simulink model "VirtualMotoTemplate"  (R2025b)
settings: Solver=daessc  StartTime=0  StopTime=2474  FixedStep=.001  RelTol=1e-2  EnableMultiTasking=on
StopFcn:
  | %toc
undefined symbols (not defined in the file): AccelOvrCmd, CtrlTcuInitGear, DecelOvrCmd, Disabled, DriverPreviewDist, EnblAccelOvr, EnblDecelCmd, EnblSteerCmd, EnvAbsPrs, EnvAirTemp, EnvGrvty, EnvNomFrictionScaling, EnvNominalGrade, EnvWindVelX, EnvWindVelY, EnvWindVelZ, FTP75, MotoFrmInert, MotoFrmLngth, MotoFrmMass, MotoLowrFrntFrkMass, MotoRearArmLngth, MotoRearArmMass, MotoUpprFrntFrkMass, RiderLkAhdPtDstGain, RiderMass, ScnAccTbl, ScnBrkTbl, ScnCRMaxLatAccel, ScnCRRadius, ScnDLCGateLongPos, ScnDLCLatRef, ScnDLCLatRefOffset, ScnDLCLongRefBpt, ScnDLCLongRefStartPos, ScnDLCVehicleWidth, ScnFHCounterDwellTime, ScnFHInitialDwellTime, ScnFHReturnTime, ScnFHRollRateZeroCross, ScnFHSteerAmp, ScnFHSteerSpeed, ScnISHandwheelRate, ScnISMaxHandwheelAng, ScnISMaxLatAccel, ScnISSteerHoldTime, ScnLongPosBpts, ScnLongVelRef, ScnOvalTrackl, ScnOvalTrackpdst, ScnOvalTrackr, ScnSDDwellTime, ScnSDSteerAmp, ScnSDSteerFreq, ScnSSFinalFreq, ScnSSSteerAmp, ScnSSSweepTime, ScnStartTime, ScnStrgAngTbl, ScnStrgTrqTbl ... (+10)
libraries: simulink x16, vehdynlibscenariocommon x9, sm_lib x6, autolibshared x4, nesl_utility x4, vehdynlibviscommon x3, sim3dgroundtruthsensorlib x2, vehdynlibdriver x2, sharedtransform x1, autolibutils x1, sim3dautolib x1, sim3dlib x1
(part 3 of 6)

== system VirtualMotoTemplate/Motorcycle Vehicle/Propulsion System/Actuators ==
  note: 1) Add Subsystem or Model blocks as valid variant choices.
      | 2) You cannot connect blocks at this level. At simulation, connectivity is automatically
      | determined, based on the active variant and port name matching.
  TrqCmd : Inport
  EngSpd : Inport  Port=2
  EMTrqCmd : Inport  Port=3
  EMSpd : Inport  Port=4
  AmbTemp : Inport  Port=5
  MotoElectricalSystem : Subsystem  VariantControl=MotoElectricalSystem  ReferencedSubsystem=MotoElectricalSystem
  MotoMappedEngine : Subsystem  VariantControl=MotoMappedEngine  ReferencedSubsystem=MotoMappedEngine
  MotoSimpleEngine : Subsystem  VariantControl=MotoSimpleEngine  ReferencedSubsystem=MotoSimpleEngine
  Eng : Outport
  Battery : Outport  Port=2
  ElecMachine : Outport  Port=3

== system VirtualMotoTemplate/Motorcycle Vehicle/Propulsion System/Electrical System Input ==
  Cntrl : Inport
  Driveline : Inport  Port=2
  Env : Inport  Port=3
  Bus Selector : BusSelector  OutputSignals=VCU.EMTrqCmd
  Bus Selector1 : BusSelector  OutputSignals=EMSpd
  Bus Selector2 : BusSelector  OutputSignals=Temp
  First Order Hold : FirstOrderHold  ErrorTolerance=inf
  EMTrqCmd : Outport  VectorParamsAs1DForOutWhenUnconnected=off
  EMSpd : Outport  Port=2  VectorParamsAs1DForOutWhenUnconnected=off
  AmbTemp : Outport  Port=3  VectorParamsAs1DForOutWhenUnconnected=off
  wires:
  Cntrl/1 -> Bus Selector/1
  Bus Selector/1 -> First Order Hold/1  "<EMTrqCmd>"
  Bus Selector1/1 -> EMSpd/1  "<EMSpd>"
  Env/1 -> Bus Selector2/1
  Bus Selector2/1 -> AmbTemp/1  "<Temp>"
  Driveline/1 -> Bus Selector1/1
  First Order Hold/1 -> EMTrqCmd/1

== system VirtualMotoTemplate/Motorcycle Vehicle/Propulsion System/Engine Input ==
  Cntrl : Inport
  Driveline : Inport  Port=2
  Bus Selector : BusSelector  OutputSignals=ECU.EngTrqCmd
  Bus Selector1 : BusSelector  OutputSignals=EngSpd
  First Order Hold : FirstOrderHold  OutputAlgorithm=Fast (Minimize Error)  ErrorTolerance=.01
  EngTrqCmd : Outport  VectorParamsAs1DForOutWhenUnconnected=off
  EngSpd : Outport  Port=2  VectorParamsAs1DForOutWhenUnconnected=off
  wires:
  Driveline/1 -> Bus Selector1/1
  Cntrl/1 -> Bus Selector/1
  Bus Selector/1 -> First Order Hold/1  "<EngTrqCmd>"
  Bus Selector1/1 -> EngSpd/1  "<EngSpd>"
  First Order Hold/1 -> EngTrqCmd/1

== system VirtualMotoTemplate/Motorcycle Vehicle/Transmission, Driveline and Brakes/Brake Hydraulics ==
  BrkPrsCmd : Inport
  Front Bias : Constant
  Gain4 : Gain  Gain=8e6
  Mux : Mux  Inputs=2
  Product : Product
  Rear Bias : Constant  Value=.6
  Valve : autolibutils/Cont LPF  wc=20*2*pi  AbsoluteTolerance=auto  aMode=2
  BrkPrs : Outport  VectorParamsAs1DForOutWhenUnconnected=off
  wires:
  Valve/1 -> Product/2
  Gain4/1 -> BrkPrs/1
  BrkPrsCmd/1 -> Valve/1
  Front Bias/1 -> Mux/1
  Rear Bias/1 -> Mux/2
  Product/1 -> Gain4/1
  Mux/1 -> Product/1

== system VirtualMotoTemplate/Motorcycle Vehicle/Transmission, Driveline and Brakes/Driveline Input ==
  Cntrl : Inport
  EngTrqCmd : Inport  Port=2
  Wheels : Inport  Port=3
  Moto : Inport  Port=4
  EMTrqCmd : Inport  Port=5
  Bus Selector : BusSelector  OutputSignals=EngTrq
  Bus Selector1 : BusSelector  OutputSignals=EMTrq
  Bus Selector2 : BusSelector  OutputSignals=RearTire.Fx,RearTire.MBrk,RearTire.Omegadot
  Bus Selector3 : BusSelector  OutputSignals=Transmission.GearCmd,VCU.VcuBrkPrsCmd
  Bus Selector5 : BusSelector  OutputSignals=Frame.Genrl.Ang.thetafrm,RearArm.Genrl.Ang.thetara
  Data Type Conversion : DataTypeConversion  SaturateOnIntegerOverflow=off  RndMeth=Floor
  First Order Hold1 : FirstOrderHold  OutputAlgorithm=Fast (Minimize Error)  ErrorTolerance=.001
  First Order Hold2 : FirstOrderHold  InitialOutput=CtrlTcuInitGear  ErrorTolerance=.5
  EngTrq : Outport  VectorParamsAs1DForOutWhenUnconnected=off
  GearCmd : Outport  Port=2  VectorParamsAs1DForOutWhenUnconnected=off
  FCpR. : Outport  Port=3  VectorParamsAs1DForOutWhenUnconnected=off
  ThetaFrm. : Outport  Port=4  VectorParamsAs1DForOutWhenUnconnected=off
  ThetaArmR. : Outport  Port=5  VectorParamsAs1DForOutWhenUnconnected=off
  MBrkR. : Outport  Port=6  VectorParamsAs1DForOutWhenUnconnected=off
  AngAWhlR. : Outport  Port=7  VectorParamsAs1DForOutWhenUnconnected=off
  EMTrq : Outport  Port=8  VectorParamsAs1DForOutWhenUnconnected=off
  BrkPrsCmd : Outport  Port=9  VectorParamsAs1DForOutWhenUnconnected=off
  wires:
  Wheels/1 -> Bus Selector2/1
  Moto/1 -> Bus Selector5/1
  Bus Selector2/3 -> AngAWhlR./1  "<Omegadot>"
  Bus Selector2/2 -> MBrkR./1  "<MBrk>"
  Bus Selector2/1 -> FCpR./1  "<Fx>"
  Bus Selector5/2 -> ThetaArmR./1  "<thetara>"
  Bus Selector5/1 -> ThetaFrm./1  "<thetafrm>"
  EngTrqCmd/1 -> Bus Selector/1
  EMTrqCmd/1 -> Bus Selector1/1
  Bus Selector3/2 -> First Order Hold1/1  "<VcuBrkPrsCmd>"
  Bus Selector3/1 -> Data Type Conversion/1  "<GearCmd>"
  Cntrl/1 -> Bus Selector3/1
  Bus Selector/1 -> EngTrq/1  "<EngTrq>"
  Bus Selector1/1 -> EMTrq/1  "<EMTrq>"
  First Order Hold1/1 -> BrkPrsCmd/1
  Data Type Conversion/1 -> First Order Hold2/1
  First Order Hold2/1 -> GearCmd/1

== system VirtualMotoTemplate/Motorcycle Vehicle/Transmission, Driveline and Brakes/Driveline Output ==
  EngSpd : Inport
  Gear : Inport  Port=2
  Info : Inport  Port=3
  EMSpd : Inport  Port=4
  BrkPrs : Inport  Port=5
  Bus Creator1 : BusCreator  Inputs=7
  Ground{,1..3} (4 alike) : Ground
  Mux : Mux  Inputs=2
  Mux1 : Mux  Inputs=2
  Signal Specification7 : SignalSpecification  Unit=Pa  Dimensions=2
  Driveline : Outport  VectorParamsAs1DForOutWhenUnconnected=off
  wires:
  Bus Creator1/1 -> Driveline/1  "Driveline"
  EngSpd/1 -> Bus Creator1/3  "EngSpd"
  EMSpd/1 -> Bus Creator1/2  "EMSpd"
  Gear/1 -> Bus Creator1/4  "Gear"
  Info/1 -> Bus Creator1/7  "Info"
  Mux/1 -> Bus Creator1/6  "AxlTrq"
  Mux1/1 -> Bus Creator1/5  "PropShftSpd"
  Ground3/1 -> Mux/2
  Ground2/1 -> Mux/1
  Ground/1 -> Mux1/1
  Ground1/1 -> Mux1/2
  BrkPrs/1 -> Signal Specification7/1
  Signal Specification7/1 -> Bus Creator1/1  "BrkPrs"

== system VirtualMotoTemplate/Motorcycle Vehicle/Transmission, Driveline and Brakes/Transmission and Driveline ==
  EngTrq : Inport
  GearCmd : Inport  Port=2
  FCpR : Inport  Port=3
  ThetaFrm : Inport  Port=4
  ThetaArmR : Inport  Port=5
  MBrkR : Inport  Port=6
  AngAWhlR : Inport  Port=7
  EMTrq : Inport  Port=8
  Driveline : Subsystem  Variant=on  VariantChoicesSpecifier={'Chain_Drive', 'No_Chain_Drive'}  VariantControlMode=label  VariantControl=Choice  LabelModeActiveChoice=Chain_Drive
  Transmission : Subsystem  Variant=on  VariantChoicesSpecifier={'ConventionalMotorcycle', 'ElectricMotorcycle'}  VariantControlMode=label  VariantControl=Choice  LabelModeActiveChoice=ConventionalMotorcycle
  EngSpd : Outport
  Gear : Outport  Port=2
  Info : Outport  Port=3
  EMSpd : Outport  Port=4
  wires:
  EngTrq/1 -> Transmission/1(EngTrq)
  GearCmd/1 -> Transmission/2(GearCmd)
  FCpR/1 -> Driveline/1(FCpR)
  ThetaFrm/1 -> Driveline/2(ThetaFrm)
  ThetaArmR/1 -> Driveline/3(ThetaArmR)
  MBrkR/1 -> Driveline/4(MBrkR)
  AngAWhlR/1 -> Driveline/5(AngAWhlR)
  EMTrq/1 -> Transmission/3(EMTrq)
  Driveline/2(DrvSprktSpd) -> Transmission/4(DrvSprktSpd)
  Transmission/4(DrvSprktTrq) -> Driveline/6(DrvSprktTrq)
  Driveline/1(Info) -> Info/1
  Transmission/1(EngSpd) -> EngSpd/1
  Transmission/2(Gear) -> Gear/1
  Transmission/3(EMSpd) -> EMSpd/1

== system VirtualMotoTemplate/Reference Generator for Motorcycle/3D Engine/3D Engine ==
  MotoFdbk : Inport
  Bus Selector1 : BusSelector  OutputSignals=Geom.FrmRotInfo
  Bus Selector2 : BusSelector  OutputSignals=Geom.posOrigin_w,Geom.posFw_l,Geom.posRw_l
  Bus Selector3 : BusSelector  OutputSignals=Geom.StrRotInfo
  Fork Translation : Constant  Value=[0 0 0]  VectorParams1D=off
  Rate Transition : RateTransition  OutPortSampleTime=dt3D
  Rotation : Concatenate  NumInputs=4  Mode=Multidimensional array
  Simulation 3D Motorcycle : sim3dautolib/Simulation 3D Motorcycle  Priority=-1  Mesh=Sports bike  MotorcycleColor=Red  ActorName=SimulinkVehicle1  MotorcycleLightsControl=off  HeadlightColor=[ 1, 1, 1 ]  HighBeamIntensity=100000  LowBeamIntensity=60000  HighBeamConeAngle=1.22  LowBeamConeAngle=1.22  HeadlightOrientation=[ 0, 0 ]  BrakelightIntensity=500  SignallightIntensity=500  SignallightPeriod=1  SignalPulseWidth=50  Translation=[X_o,Y_o,Z_o; zeros(3, 3 )]  Rotation=[phi_o,theta_o, psi_o;zeros(3, 3 )]  SampleTime=dt3D  ActorType=SimulinkVehicle  ID=1  aMode=2  ActorTag=SimulinkVehicle1
  Simulation 3D Scene Configuration : sim3dlib/Simulation 3D Scene Configuration  Priority=0  ProjectFormat=Default Scenes  SceneDesc=Open surface  ProjectName=/mathworks/devel/bat/filer/batfs2552-0/BR2025bd.3077943.BR2025bd.3070728.pass/build/matlab/toolbox/shared/sim3d_projects/automotive_project_linux/UE/LinuxNoEditor/VehicleSimulation.sh  ScenePath=/Game/Maps/HwStrght  EnableOpenDRIVE=off  vehTagList={'Custom';'Scene Origin';'SimulinkVehicle1'}  vehTag=SimulinkVehicle1  AttachedCameraRelativeTranslation=[0 0 0]  FreeCameraDefaultInitialTranslation=[-6, 0, 2]  AttachedCameraRelativeRotation=[0, -15, 0]  FreeCameraDefaultInitialRotation=[0, -15, 0]  ViewpointName=Custom  FreeCameraInitialTranslation=[0 0 0]  ViewpointTranslation=[0 0 0]  FreeCameraInitialRotation=[0 0 0]  ViewpointRotation=[0 0 0]  OpVisEn=off  Ts=dt3D  EnableWindow=on  EnableRemoteAccess=off  EnableWeather=off  SunAzimuth=180  SunAltitude=60  EnableGeospatialSun=off  Latitude=0  Longitude=0  Date=2023-01-01  Time=10:30:00  GeoTimeZone=-5.0  SunDaylightSaving=off  wind=1  clouds=40  EnableVolumetricClouds=off  CloudCoverage=0  CloudAltitude=6  fog=0.0  rain=0.0  RaindropsEffect=off  SnowDensity=0  EnableGeospatial=off  TilesetSource=Earth terrain  UseTrueOrigin=off  OriginHeight=200  OriginLatitude=40.744652  OriginLongitude=-73.988864  MapStyle=Aerial  AdditionalAssetIDs=[]  UseAdvancedSunSky=off  SolarTime=11  TimeZone=-5  Day=21  Month=9  Year=2022  UseDaylightSavingTime=on  DSTStartDay=10  DSTStartMonth=3  DSTEndDay=3  DSTEndMonth=11  DSTSwitchHour=2  sensorTag=MainCamera1  sensorId=1  sensorName=MainCamera1  mountLoc=Origin  offsetFlag=off  tmountOffset=[0, 0, 0]  rmountOffset=[0, 0, 0]  HorizontalResolution=1280  VerticalResolution=720  HorizontalFOV=60  mountPoint=[0 0 0]  mountOrientation=[0 0 0]  aMode=aMode  ID=1  GeoTrigger=Inactive  ViewNameList={'Custom'}  ViewTranslationList={'[0 0 0]'}  ViewRotationList={'[0 0 0]'}
  Translation : Concatenate  NumInputs=4  Mode=Multidimensional array
  Wheel Rotations : Subsystem
  wires:
  Wheel Rotations/2(Rear) -> Rotation/4
  Bus Selector1/1 -> Rotation/1  "<FrmRotInfo>"
  Rotation/1 -> Simulation 3D Motorcycle/2
  Translation/1 -> Simulation 3D Motorcycle/1
  Fork Translation/1 -> Translation/2
  Bus Selector2/1 -> Translation/1  "<posOrigin_w>"
  Bus Selector3/1 -> Rotation/2  "<StrRotInfo>"
  Wheel Rotations/1(Front) -> Rotation/3
  Bus Selector2/3 -> Translation/4  "<posRw_l>"
  Rate Transition/1 -> Bus Selector2/1, Wheel Rotations/1(MotoFdbk), Bus Selector3/1, Bus Selector1/1
  MotoFdbk/1 -> Rate Transition/1
  Bus Selector2/2 -> Translation/3  "<posFw_l>"

== system VirtualMotoTemplate/Reference Generator for Motorcycle/3D Engine/3D Engine Disabled ==
  MotoFdbk : Inport
  Terminator : Terminator
  wires:
  MotoFdbk/1 -> Terminator/1

== system VirtualMotoTemplate/Reference Generator for Motorcycle/Reference Generator/Double Lane Change ==
  "MotoFdbk " : Inport
  Double Lane Change : vehdynlibscenariocommon/Lane Change Reference Generator  VariantControl=Variant1  ssMode=Initialize from model  ssVar=dlcSS35mph  changeType=Obstacle avoidance (ISO 3888-2)  t_start=t_start  XGate=XGate  xdot_r=xdot_r  xdotUnit=mph  xStart=xStart  vehW=vehW  latoff=latoff  lattoff=VEH.InitialLatPosition  centerSwitch=on  xSimStop=off  ssDefault=off  latRefbp=latRefbp  latRef=latRef  X_o=X_o  Y_o=Y_o  psi_o=phi_o  ssTol=1e-3  ssMaxTime=30  ssWSName=dlcSS35mph  aMode=2  use3DCones=off
  " Vis" : Outport  VectorParamsAs1DForOutWhenUnconnected=off
  " Ref" : Outport  Port=2  VectorParamsAs1DForOutWhenUnconnected=off
  " Fdbk" : Outport  Port=3  VectorParamsAs1DForOutWhenUnconnected=off
  wires:
  "MotoFdbk "/1 -> " Fdbk"/1, Double Lane Change/1
  Double Lane Change/1 -> " Vis"/1
  Double Lane Change/2 -> " Ref"/1

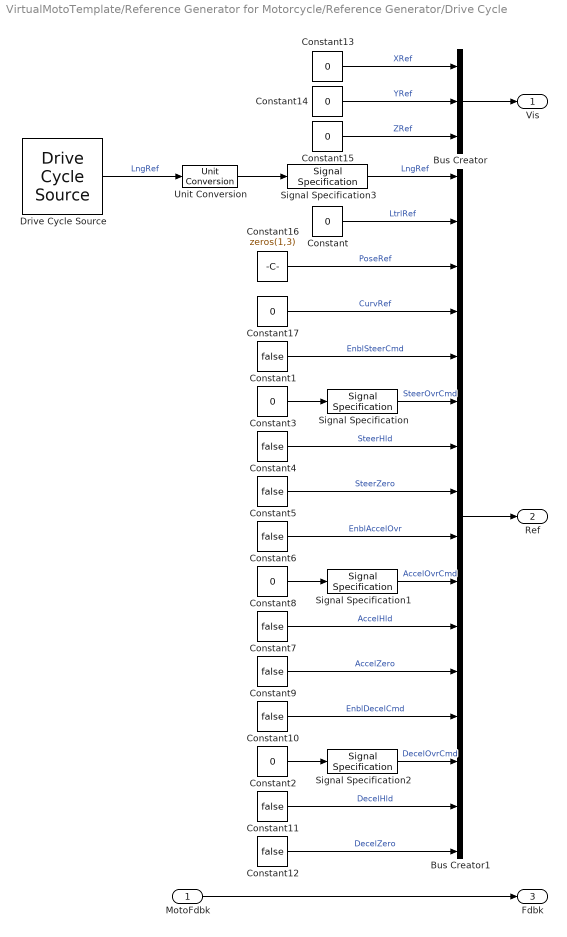
== system VirtualMotoTemplate/Reference Generator for Motorcycle/Reference Generator/Drive Cycle ==
  "MotoFdbk " : Inport
  Bus Creator : BusCreator  Inputs=3
  Bus Creator1 : BusCreator  Inputs=16
  Constant{,2..3,8,13..15,17} (8 alike) : Constant  Value=0
  Constant{1,4..7,9..12} (9 alike) : Constant  Value=false
  Constant16 : Constant  Value=zeros(1,3)
  Drive Cycle Source : autolibshared/Drive Cycle Source  cycleVar=FTP75  fileVar=L:\Bauto\matlab\test\toolbox\shared\autoblks\scenario\adac.txt  tfinal="2474  seconds"  cycleRepeat=off  outAccPort=off  outGearPort=off  gearList=No gear data  t_wot1=ScnStartTime  xdot_woto=0  xdot_wot1=ScnLongVelRef  t_wot2=ScnTimeToStrtDecel  xdot_wot2=0  t_wotend=ScnSimTime  srcUnit=m/s  outUnit=mph  srcAccUnit=m/s/s  outAccUnit=m/s^2  dt=0  aMode=6  faultOption=off  velBnd=2  velBndUnit=mph  inUnit=m/s  timeBnd=1  failOption=off  stopSim=off  maxFaultCnt=10  maxFaultTime=2  maxTotFaultTime=15  traceOption=off  dtTrace=1  traceWindow=10  lastDCname=FTP75  lastOutUnit=mph  lastDT=0  lastTB=1  lastSB=2  forceCalcBound=off
  Signal Specification : SignalSpecification  Unit=rad
  Signal Specification1 : SignalSpecification  Unit=one
  Signal Specification2 : SignalSpecification  Unit=one
  Signal Specification3 : SignalSpecification  Unit=m/s
  Unit Conversion : UnitConversion
  " Vis" : Outport  VectorParamsAs1DForOutWhenUnconnected=off
  " Ref" : Outport  Port=2  VectorParamsAs1DForOutWhenUnconnected=off
  " Fdbk" : Outport  Port=3  VectorParamsAs1DForOutWhenUnconnected=off
  wires:
  Constant2/1 -> Signal Specification2/1
  Constant8/1 -> Signal Specification1/1
  Constant4/1 -> Bus Creator1/7  "SteerHld"
  Signal Specification2/1 -> Bus Creator1/14  "DecelOvrCmd"
  Constant12/1 -> Bus Creator1/16  "DecelZero"
  Constant6/1 -> Bus Creator1/9  "EnblAccelOvr"
  Constant7/1 -> Bus Creator1/11  "AccelHld"
  Constant9/1 -> Bus Creator1/12  "AccelZero"
  Signal Specification1/1 -> Bus Creator1/10  "AccelOvrCmd"
  Constant11/1 -> Bus Creator1/15  "DecelHld"
  Constant10/1 -> Bus Creator1/13  "EnblDecelCmd"
  Constant5/1 -> Bus Creator1/8  "SteerZero"
  Signal Specification/1 -> Bus Creator1/6  "SteerOvrCmd"
  Constant3/1 -> Signal Specification/1
  Constant1/1 -> Bus Creator1/5  "EnblSteerCmd"
  Constant/1 -> Bus Creator1/2  "LtrlRef"
  Signal Specification3/1 -> Bus Creator1/1  "LngRef"
  Bus Creator1/1 -> " Ref"/1
  "MotoFdbk "/1 -> " Fdbk"/1
  Bus Creator/1 -> " Vis"/1
  Constant15/1 -> Bus Creator/3  "ZRef"
  Constant14/1 -> Bus Creator/2  "YRef"
  Constant13/1 -> Bus Creator/1  "XRef"
  Constant16/1 -> Bus Creator1/3  "PoseRef"
  Constant17/1 -> Bus Creator1/4  "CurvRef"
  Drive Cycle Source/1 -> Unit Conversion/1  "LngRef"
  Unit Conversion/1 -> Signal Specification3/1

== system VirtualMotoTemplate/Reference Generator for Motorcycle/Reference Generator/Fishhook ==
  "MotoFdbk " : Inport
  Bus Creator : BusCreator  Inputs=3
  Constant : Constant  Value=0
  Constant1 : Constant  Value=0
  Constant2 : Constant  Value=0
  Fishhook : vehdynlibscenariocommon/Fishhook  ssMode=Initialize from model  ssVar=fh50mph  t_start=t_start  xdot_r=xdot_r  xdotUnit=mph  steerRate=steerRate  steerA=steerAFH  pFdbk=off  tDwell1=tDwell1  tDwell2=tDwell2  tSteer3=tSteer3  pZero=pZero  steerDir=off  ssDefault=off  X_o=0  Y_o=0  psi_o=0  ssTol=1  ssMaxTime=30  ssWSName=fh50mph  aMode=2
  " Vis" : Outport  VectorParamsAs1DForOutWhenUnconnected=off
  " Ref" : Outport  Port=2  VectorParamsAs1DForOutWhenUnconnected=off
  " Fdbk" : Outport  Port=3  VectorParamsAs1DForOutWhenUnconnected=off
  wires:
  Constant/1 -> Bus Creator/1  "XRef"
  Constant1/1 -> Bus Creator/2  "YRef"
  Constant2/1 -> Bus Creator/3  "ZRef"
  Bus Creator/1 -> " Vis"/1
  Fishhook/1 -> " Ref"/1
  "MotoFdbk "/1 -> " Fdbk"/1, Fishhook/1

== system VirtualMotoTemplate/Reference Generator for Motorcycle/Reference Generator/Increasing Steer ==
  "MotoFdbk " : Inport
  Bus Creator : BusCreator  Inputs=3
  Constant : Constant  Value=0
  Constant1 : Constant  Value=0
  Constant2 : Constant  Value=0
  Increasing Steer : vehdynlibscenariocommon/Slowly Increasing Steer  VariantControl=1  ssMode=Initialize from model  ssVar=is50mph  t_start=t_start  xdot_r=xdot_r  xdotUnit=mph  omega_hw=omega_hw  theta_max=theta_max  t_stop=t_stop  ay_max=ay_max  steerDir=off  ay_stop=off  ssDefault=off  X_o=0  Y_o=0  psi_o=0  ssTol=1  ssMaxTime=30  ssWSName=is50mph  aMode=2
  " Vis" : Outport  VectorParamsAs1DForOutWhenUnconnected=off
  " Ref" : Outport  Port=2  VectorParamsAs1DForOutWhenUnconnected=off
  " Fdbk" : Outport  Port=3  VectorParamsAs1DForOutWhenUnconnected=off
  wires:
  "MotoFdbk "/1 -> " Fdbk"/1, Increasing Steer/1
  Bus Creator/1 -> " Vis"/1
  Increasing Steer/1 -> " Ref"/1
  Constant2/1 -> Bus Creator/3  "ZRef"
  Constant1/1 -> Bus Creator/2  "YRef"
  Constant/1 -> Bus Creator/1  "XRef"

== system VirtualMotoTemplate/Reference Generator for Motorcycle/Reference Generator/Longitudinal Maneuver Tracking ==
  "MotoFdbk " : Inport
  Bus Creator : BusCreator  Inputs=3
  Bus Creator1 : BusCreator  Inputs=14
  Constant{,2..3,8} (4 alike) : Constant  Value=0
  Constant{1,4..7,9..12} (9 alike) : Constant  Value=false
  Constant13 : Constant  Value=xdot_r
  Ground : Ground
  Ground1 : Ground
  Ground2 : Ground
  Signal Specification1 : SignalSpecification  Unit=one
  Signal Specification2 : SignalSpecification  Unit=one
  Signal Specification3 : SignalSpecification  Unit=m/s
  Unit Conversion : UnitConversion
  refUnit : SignalSpecification  Unit=mph  mask{Unit=mph}
      mask prompts: Unit "Simulink:blkprm_prompts:OutputUnit_EditField"
      mask TypeOptions Unit: Unit
      mask DialogControl Unit Prompt: Unit (e.g., m, m/s^2, N*m):
  " Vis" : Outport
  " Ref" : Outport  Port=2
  " Fdbk" : Outport  Port=3
  wires:
  Ground/1 -> Bus Creator/1  "XRef"
  Ground2/1 -> Bus Creator/3  "ZRef"
  Constant6/1 -> Bus Creator1/7  "EnblAccelOvr"
  Constant/1 -> Bus Creator1/2  "LtrlRef"
  Bus Creator1/1 -> " Ref"/1
  Constant5/1 -> Bus Creator1/6  "SteerZero"
  Constant7/1 -> Bus Creator1/9  "AccelHld"
  Signal Specification1/1 -> Bus Creator1/8  "AccelOvrCmd"
  Ground1/1 -> Bus Creator/2  "YRef"
  Constant3/1 -> Bus Creator1/4  "SteerOvrCmd"
  Bus Creator/1 -> " Vis"/1
  Constant12/1 -> Bus Creator1/14  "DecelZero"
  Constant1/1 -> Bus Creator1/3  "EnblSteerCmd"
  Constant10/1 -> Bus Creator1/11  "EnblDecelCmd"
  Constant11/1 -> Bus Creator1/13  "DecelHld"
  Signal Specification2/1 -> Bus Creator1/12  "DecelOvrCmd"
  Constant2/1 -> Signal Specification2/1
  Constant8/1 -> Signal Specification1/1
  Constant4/1 -> Bus Creator1/5  "SteerHld"
  Constant9/1 -> Bus Creator1/10  "AccelZero"
  "MotoFdbk "/1 -> " Fdbk"/1
  Signal Specification3/1 -> Bus Creator1/1  "LngRef"
  Constant13/1 -> refUnit/1
  Unit Conversion/1 -> Signal Specification3/1
  refUnit/1 -> Unit Conversion/1

== system VirtualMotoTemplate/Reference Generator for Motorcycle/Reference Generator/Manual Maneuver Design ==
  "MotoFdbk " : Inport
  Bus Creator : BusCreator  Inputs=3
  Bus Creator1 : BusCreator  Inputs=16
  Constant{,1..3,5..6,14,17..18} (9 alike) : Constant  Value=0
  Constant{4,7..13,15} (9 alike) : Constant  Value=false
  Constant16 : Constant  Value=zeros(1,3)
  Signal Specification : SignalSpecification  Unit=rad
  Signal Specification1 : SignalSpecification  Unit=one
  Signal Specification2 : SignalSpecification  Unit=one
  " Vis" : Outport  VectorParamsAs1DForOutWhenUnconnected=off
  " Ref" : Outport  Port=2  VectorParamsAs1DForOutWhenUnconnected=off
  " Fdbk" : Outport  Port=3  VectorParamsAs1DForOutWhenUnconnected=off
  wires:
  "MotoFdbk "/1 -> " Fdbk"/1
  Constant2/1 -> Bus Creator/3  "ZRef"
  Constant/1 -> Bus Creator/1  "XRef"
  Constant1/1 -> Bus Creator/2  "YRef"
  Bus Creator/1 -> " Vis"/1
  Bus Creator1/1 -> " Ref"/1
  Constant16/1 -> Bus Creator1/3  "PoseRef"
  Constant3/1 -> Bus Creator1/2  "LtrlRef"
  Constant10/1 -> Bus Creator1/13  "EnblDecelCmd"
  Constant17/1 -> Bus Creator1/4  "CurvRef"
  Constant18/1 -> Bus Creator1/1  "LngRef"
  Constant8/1 -> Bus Creator1/8  "SteerZero"
  Constant5/1 -> Signal Specification2/1
  Constant7/1 -> Bus Creator1/7  "SteerHld"
  Signal Specification1/1 -> Bus Creator1/10  "AccelOvrCmd"
  Signal Specification2/1 -> Bus Creator1/14  "DecelOvrCmd"
  Constant12/1 -> Bus Creator1/16  "DecelZero"
  Constant9/1 -> Bus Creator1/9  "EnblAccelOvr"
  Constant15/1 -> Bus Creator1/12  "AccelZero"
  Constant14/1 -> Signal Specification1/1
  Constant4/1 -> Bus Creator1/5  "EnblSteerCmd"
  Signal Specification/1 -> Bus Creator1/6  "SteerOvrCmd"
  Constant6/1 -> Signal Specification/1
  Constant11/1 -> Bus Creator1/15  "DecelHld"
  Constant13/1 -> Bus Creator1/11  "AccelHld"

== system VirtualMotoTemplate/Reference Generator for Motorcycle/Reference Generator/Sine with Dwell ==
  "MotoFdbk " : Inport
  Bus Creator : BusCreator  Inputs=3
  Constant : Constant  Value=0
  Constant1 : Constant  Value=0
  Constant2 : Constant  Value=0
  Sine With Dwell : vehdynlibscenariocommon/Sine With Dwell  VariantControl=3  ssMode=Initialize from model  ssVar=swd50mph  t_start=t_start  xdot_r=xdot_r  xdotUnit=mph  steerF=steerF  steerA=steerA  tdwell=tdwell  steerDir=off  ssDefault=off  X_o=0  Y_o=0  psi_o=0  ssTol=1  ssMaxTime=30  ssWSName=swd50mph  aMode=2
  " Vis" : Outport  VectorParamsAs1DForOutWhenUnconnected=off
  " Ref" : Outport  Port=2  VectorParamsAs1DForOutWhenUnconnected=off
  " Fdbk" : Outport  Port=3  VectorParamsAs1DForOutWhenUnconnected=off
  wires:
  Sine With Dwell/1 -> " Ref"/1
  "MotoFdbk "/1 -> " Fdbk"/1, Sine With Dwell/1
  Bus Creator/1 -> " Vis"/1
  Constant2/1 -> Bus Creator/3  "ZRef"
  Constant1/1 -> Bus Creator/2  "YRef"
  Constant/1 -> Bus Creator/1  "XRef"

== system VirtualMotoTemplate/Reference Generator for Motorcycle/Reference Generator/Swept Sine ==
  "MotoFdbk " : Inport
  Bus Creator : BusCreator  Inputs=3
  Constant : Constant  Value=0
  Constant1 : Constant  Value=0
  Constant2 : Constant  Value=0
  Swept Sine : vehdynlibscenariocommon/Swept Sine Reference Generator  VariantControl=2  ssMode=Initialize from model  ssVar=ss30mph  t_start=t_start  xdot_r=xdot_r  xdotUnit=mph  theta_hw=theta_hw  theta_hw_final=theta_hw_final  t_sweep=t_sweep  ssDefault=off  X_o=0  Y_o=0  psi_o=0  ssTol=1  ssMaxTime=30  ssWSName=ss30mph  aMode=2
  " Vis" : Outport  VectorParamsAs1DForOutWhenUnconnected=off
  " Ref" : Outport  Port=2  VectorParamsAs1DForOutWhenUnconnected=off
  " Fdbk" : Outport  Port=3  VectorParamsAs1DForOutWhenUnconnected=off
  wires:
  "MotoFdbk "/1 -> " Fdbk"/1, Swept Sine/1
  Swept Sine/1 -> " Ref"/1
  Bus Creator/1 -> " Vis"/1
  Constant2/1 -> Bus Creator/3  "ZRef"
  Constant1/1 -> Bus Creator/2  "YRef"
  Constant/1 -> Bus Creator/1  "XRef"

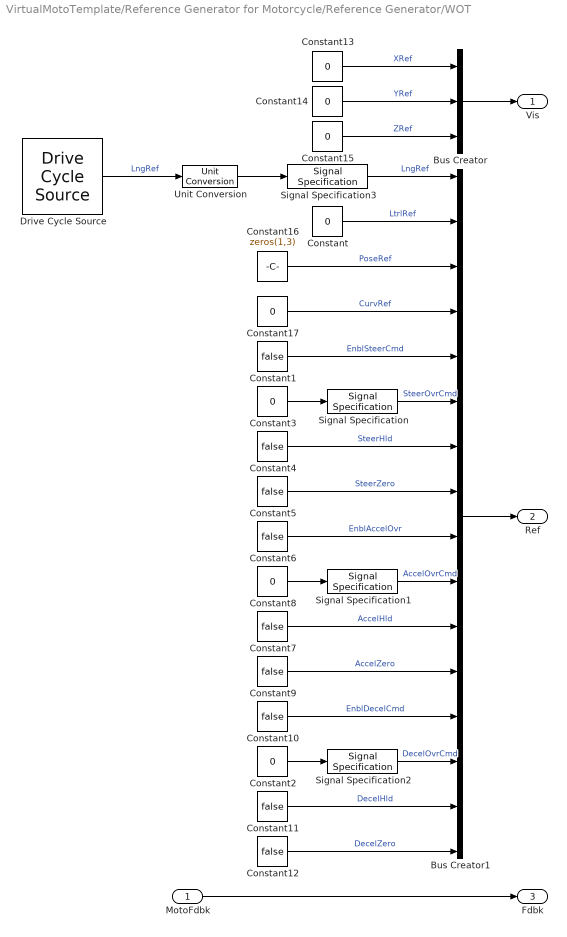
== system VirtualMotoTemplate/Reference Generator for Motorcycle/Reference Generator/WOT ==
  "MotoFdbk " : Inport
  Bus Creator : BusCreator  Inputs=3
  Bus Creator1 : BusCreator  Inputs=16
  Constant{,2..3,8,13..15,17} (8 alike) : Constant  Value=0
  Constant{1,4..7,9..12} (9 alike) : Constant  Value=false
  Constant16 : Constant  Value=zeros(1,3)
  Drive Cycle Source : autolibshared/Drive Cycle Source  cycleVar=Wide Open Throttle (WOT)  fileVar=L:\Bauto\matlab\test\toolbox\shared\autoblks\scenario\adac.txt  tfinal="40  seconds"  cycleRepeat=off  outAccPort=off  outGearPort=off  gearList=No gear data  t_wot1=ScnStartTime  xdot_woto=0  xdot_wot1=xdot_wot1  t_wot2=t_wot2  xdot_wot2=0  t_wotend=ScnSimTime  srcUnit=mph  outUnit=mph  srcAccUnit=m/s/s  outAccUnit=m/s^2  dt=0  aMode=6  faultOption=off  velBnd=2  velBndUnit=mph  inUnit=m/s  timeBnd=1  failOption=off  stopSim=off  maxFaultCnt=10  maxFaultTime=2  maxTotFaultTime=15  traceOption=off  dtTrace=1  traceWindow=10  lastDCname=Custom Data Set  lastOutUnit=mph  lastDT=0  lastTB=1  lastSB=2  forceCalcBound=off
  Signal Specification : SignalSpecification  Unit=rad
  Signal Specification1 : SignalSpecification  Unit=one
  Signal Specification2 : SignalSpecification  Unit=one
  Signal Specification3 : SignalSpecification  Unit=m/s
  Unit Conversion : UnitConversion
  " Vis" : Outport  VectorParamsAs1DForOutWhenUnconnected=off
  " Ref" : Outport  Port=2  VectorParamsAs1DForOutWhenUnconnected=off
  " Fdbk" : Outport  Port=3  VectorParamsAs1DForOutWhenUnconnected=off
  wires:
  Constant2/1 -> Signal Specification2/1
  Constant8/1 -> Signal Specification1/1
  Constant4/1 -> Bus Creator1/7  "SteerHld"
  Signal Specification2/1 -> Bus Creator1/14  "DecelOvrCmd"
  Constant12/1 -> Bus Creator1/16  "DecelZero"
  Constant6/1 -> Bus Creator1/9  "EnblAccelOvr"
  Constant7/1 -> Bus Creator1/11  "AccelHld"
  Constant9/1 -> Bus Creator1/12  "AccelZero"
  Signal Specification1/1 -> Bus Creator1/10  "AccelOvrCmd"
  Constant11/1 -> Bus Creator1/15  "DecelHld"
  Constant10/1 -> Bus Creator1/13  "EnblDecelCmd"
  Constant5/1 -> Bus Creator1/8  "SteerZero"
  Signal Specification/1 -> Bus Creator1/6  "SteerOvrCmd"
  Constant3/1 -> Signal Specification/1
  Constant1/1 -> Bus Creator1/5  "EnblSteerCmd"
  Constant/1 -> Bus Creator1/2  "LtrlRef"
  Signal Specification3/1 -> Bus Creator1/1  "LngRef"
  Bus Creator1/1 -> " Ref"/1
  "MotoFdbk "/1 -> " Fdbk"/1
  Bus Creator/1 -> " Vis"/1
  Constant15/1 -> Bus Creator/3  "ZRef"
  Constant14/1 -> Bus Creator/2  "YRef"
  Constant13/1 -> Bus Creator/1  "XRef"
  Constant16/1 -> Bus Creator1/3  "PoseRef"
  Constant17/1 -> Bus Creator1/4  "CurvRef"
  Drive Cycle Source/1 -> Unit Conversion/1  "LngRef"
  Unit Conversion/1 -> Signal Specification3/1

== system VirtualMotoTemplate/Reference Generator for Motorcycle/Reference Router/Maneuver Tracking ==
  VisIn : Inport
  RefIn : Inport  Port=2
  FdbkIn : Inport  Port=3
  Vis : Outport
  Ref : Outport  Port=2
  Fdbk : Outport  Port=3
  wires:
  VisIn/1 -> Vis/1
  FdbkIn/1 -> Fdbk/1
  RefIn/1 -> Ref/1

== system VirtualMotoTemplate/Reference Generator for Motorcycle/Reference Router/Steering Command Override ==
  VisIn : Inport
  RefIn : Inport  Port=2
  FdbkIn : Inport  Port=3
  Bus Assignment : BusAssignment  AssignedSignals=SteerOvrCmd,EnblSteerCmd
  Bus Selector : BusSelector  OutputSignals=Body.InertFrm.Cg.Disp.X
  Clock : Clock
  Constant : Constant  Value=true
  Control Signals : Subsystem  Variant=on
  Vis : Outport
  Ref : Outport  Port=2
  Fdbk : Outport  Port=3
  wires:
  VisIn/1 -> Vis/1
  FdbkIn/1 -> Bus Selector/1, Fdbk/1
  Clock/1 -> Control Signals/1(Time)
  Control Signals/1(Steer) -> Bus Assignment/2  "Steer"
  Bus Selector/1 -> Control Signals/2(Position)  "<X>"
  RefIn/1 -> Bus Assignment/1
  Bus Assignment/1 -> Ref/1
  Constant/1 -> Bus Assignment/3

== system VirtualMotoTemplate/Reference Generator for Motorcycle/Reference Router/Steering and Accel and Brk Command Override ==
  VisIn : Inport
  RefIn : Inport  Port=2
  FdbkIn : Inport  Port=3
  Bus Assignment : BusAssignment  AssignedSignals=SteerOvrCmd,AccelOvrCmd,DecelOvrCmd,EnblSteerCmd,EnblAccelOvr,EnblDecelCmd
  Bus Selector : BusSelector  OutputSignals=Body.InertFrm.Cg.Disp.X
  Clock : Clock
  Constant : Constant  Value=true
  Constant1 : Constant  Value=true
  Constant2 : Constant  Value=true
  Control Signals : Subsystem  Variant=on
  Vis : Outport
  Ref : Outport  Port=2
  Fdbk : Outport  Port=3
  wires:
  VisIn/1 -> Vis/1
  FdbkIn/1 -> Bus Selector/1, Fdbk/1
  Clock/1 -> Control Signals/1(Time)
  Control Signals/1(Steer) -> Bus Assignment/2  "Steer"
  Control Signals/2(Accel) -> Bus Assignment/3  "Accel"
  Control Signals/3(Brake) -> Bus Assignment/4  "Brake"
  Bus Selector/1 -> Control Signals/2(Position)  "<X>"
  RefIn/1 -> Bus Assignment/1
  Bus Assignment/1 -> Ref/1
  Constant/1 -> Bus Assignment/5
  Constant1/1 -> Bus Assignment/6
  Constant2/1 -> Bus Assignment/7

== system VirtualMotoTemplate/Rider Commands/Rider Commands/Longitudinal Rider ==
  MotoRef : Inport
  MotoFdbk : Inport  Port=2
  Env : Inport  Port=3
  Bus Creator1 : BusCreator  Inputs=5
  Bus Selector1 : BusSelector  OutputSignals=SteerOvrCmd,LngRef,EnblAccelOvr,AccelOvrCmd,AccelHld,AccelZero,EnblDecelCmd,DecelOvrCmd,DecelHld,DecelZero
  Constant : Constant  Value=false
  Equal Front Rear Bias : Selector  InputPortWidth=1  IndexOptions=Index vector (dialog)  Indices=[1 1]  OutputSizes=1
  Gain : Gain
  Hill Hold : Subsystem
  Longitudinal Driver : autolibshared/Longitudinal Driver  extAccelOvr=on  extDecelOvr=on  extAccelHld=on  extDecelHld=on  extAccelZero=on  extDecelZero=on  cntrlType=Predictive  shftType=Scheduled  velUnits=m/s  gearOut=on  Kp=5  Ki=5  Kff=.1  Kg=0  VehVelVec=[0 100]  KffVec=[.1 .1]  KpVec=[10 10]  KiVec=[5 5]  KgVec=[0 0]  m=MotoFrmMass+MotoUpprFrntFrkMass+MotoLowrFrntFrkMass+MotoRearArmMass+RiderMass  Kpt=DriverTractiveForce  tau=DriverTimeConst  L=DriverPreviewDist  aR=DriverRollRes  bR=DriverDrivelineRes  cR=DriverAeroRes  g=EnvGrvty  vnom=5  Kaw=1  tauerr=.1  tauPt=2  GearInit=DriverInitialGear  tShift=DriverShiftTime  pdlVec=[0.1 0.4 0.5 0.9]  upShftTbl=|  dwnShftTbl=|  tClutch=.5  tRev=.5  tPark=120  aMode=6  UpGearVec="[0  1  2  3  4  5  6  7  8]"  DownGearVec="[1  2  3  4  5  6  7  8  9]"
      upShftTbl=|
      | [-1 25 42.7198903036173	47.4101666153559	56.5501922484876	82.5161741607935	103.519768418748	161.279652628121	247.919478942182;
      | -1 35 47.2198903036173	51.9101666153559	61.0501922484876	87.0161741607935	108.019768418748	165.779652628121	252.419478942182;
      | -1 40 48.7198903036173	53.4101666153559	62.5501922484876	88.5161741607935	109.519768418748	167.279652628121	253.919478942182;
      | -1 45 54.7198903036173	59.4101666153559	68.5501922484876	94.5161741607935	115.519768418748	173.279652628121	259.919478942182].*0.277778
      dwnShftTbl=|
      | [6 20 38.7198903036173	43.4101666153559	52.5501922484876	78.5161741607935	99.5197684187476	157.279652628121	243.919478942182;
      | 6 30 43.2198903036173	47.9101666153559	57.0501922484876	83.0161741607935	104.019768418748	161.779652628121	248.419478942182;
      | 6 35 44.7198903036173	49.4101666153559	58.5501922484876	84.5161741607935	105.519768418748	163.279652628121	249.919478942182;
      | 6 45 50.7198903036173	55.4101666153559	64.5501922484876	90.5161741607935	111.519768418748	169.279652628121	255.919478942182].*0.277778
  Signal Specification4 : SignalSpecification  Unit=N*m
  Terminator3 : Terminator
  Unit Conversion1 : UnitConversion
  Rider : Outport  VectorParamsAs1DForOutWhenUnconnected=off
  wires:
  Bus Creator1/1 -> Rider/1
  Signal Specification4/1 -> Bus Creator1/1  "SteerCmd"
  Longitudinal Driver/3 -> Equal Front Rear Bias/1
  Longitudinal Driver/1 -> Terminator3/1
  Bus Selector1/2 -> Unit Conversion1/1  "<LngRef>"
  MotoRef/1 -> Bus Selector1/1
  MotoFdbk/1 -> Hill Hold/7(VehFdbk)
  Longitudinal Driver/2 -> Bus Creator1/2  "AccelCmd"
  Longitudinal Driver/4 -> Bus Creator1/4  "GearCmd"
  Bus Selector1/1 -> Gain/1  "<SteerOvrCmd>"
  Constant/1 -> Bus Creator1/5  "IgnSwtch"
  Bus Selector1/3 -> Longitudinal Driver/2  "<EnblAccelOvr>"
  Bus Selector1/4 -> Longitudinal Driver/3  "<AccelOvrCmd>"
  Bus Selector1/5 -> Longitudinal Driver/4  "<AccelHld>"
  Bus Selector1/6 -> Longitudinal Driver/5  "<AccelZero>"
  Bus Selector1/7 -> Hill Hold/2(<EnblDecelCmd>)  "<EnblDecelCmd>"
  Bus Selector1/8 -> Hill Hold/3(<DecelOvrCmd>)  "<DecelOvrCmd>"
  Bus Selector1/9 -> Hill Hold/4(<DecelHld>)  "<DecelHld>"
  Bus Selector1/10 -> Hill Hold/5(<DecelZero>)  "<DecelZero>"
  Hill Hold/2(DecelOvrCmd) -> Longitudinal Driver/7
  Hill Hold/1(EnblDecelOvr) -> Longitudinal Driver/6
  Hill Hold/6(Grade) -> Longitudinal Driver/11
  Env/1 -> Hill Hold/6(Env)
  Hill Hold/5(VelFdbk) -> Longitudinal Driver/10
  Hill Hold/3(DecelHld) -> Longitudinal Driver/8
  Hill Hold/4(DecelZero) -> Longitudinal Driver/9
  Unit Conversion1/1 -> Longitudinal Driver/1, Hill Hold/1(LngRef)
  Equal Front Rear Bias/1 -> Bus Creator1/3  "DecelCmd"
  Gain/1 -> Signal Specification4/1

== system VirtualMotoTemplate/Rider Commands/Rider Commands/Open Loop ==
  MotoFdbk : Inport
  MotoRef : Inport  Port=2
  GearCmd : Inport  Port=3
  Bus Creator1 : BusCreator  Inputs=5
  Bus Selector1 : BusSelector  OutputSignals=SteerOvrCmd,AccelOvrCmd,DecelOvrCmd
  Constant : Constant  Value=false
  Equal Front Rear Bias : Selector  InputPortWidth=1  IndexOptions=Index vector (dialog)  Indices=[1 1]  OutputSizes=1
  Gain : Gain
  Signal Specification : SignalSpecification  Unit=1
  Signal Specification1 : SignalSpecification  Unit=1
  Signal Specification2 : SignalSpecification  Unit=1
  Signal Specification3 : SignalSpecification  Unit=rad
  Signal Specification4 : SignalSpecification  Unit=N*m
  Terminator : Terminator
  Rider : Outport  VectorParamsAs1DForOutWhenUnconnected=off
  wires:
  Signal Specification2/1 -> Bus Creator1/4  "GearCmd"
  Bus Selector1/3 -> Signal Specification1/1  "<DecelOvrCmd>"
  Bus Creator1/1 -> Rider/1
  Bus Selector1/2 -> Signal Specification/1  "<AccelOvrCmd>"
  MotoFdbk/1 -> Terminator/1
  Signal Specification/1 -> Bus Creator1/2  "AccelCmd"
  Equal Front Rear Bias/1 -> Bus Creator1/3  "DecelCmd"
  Constant/1 -> Bus Creator1/5  "IgnSwtch"
  MotoRef/1 -> Bus Selector1/1
  GearCmd/1 -> Signal Specification2/1
  Bus Selector1/1 -> Signal Specification3/1  "<SteerOvrCmd>"
  Signal Specification4/1 -> Bus Creator1/1  "SteerCmd"
  Signal Specification1/1 -> Equal Front Rear Bias/1  "DecelCmd"
  Signal Specification3/1 -> Gain/1
  Gain/1 -> Signal Specification4/1

== system VirtualMotoTemplate/Rider Commands/Rider Commands/Predictive Rider ==
  MotoRef : Inport
  MotoFdbk : Inport  Port=2
  Env : Inport  Port=3
  Bus Creator1 : BusCreator  Inputs=5
  Bus Selector : BusSelector  OutputSignals=Body.InertFrm.Cg.Disp.Y,Body.BdyFrm.Cg.Vel.ydot,Body.InertFrm.Cg.Ang.psi,Body.BdyFrm.Cg.AngVel.r
  Bus Selector1 : BusSelector  OutputSignals=LngRef,LtrlRef,EnblSteerCmd,SteerOvrCmd,SteerHld,SteerZero,EnblAccelOvr,AccelOvrCmd,AccelHld,AccelZero,EnblDecelCmd,DecelOvrCmd,DecelHld,DecelZero
  Constant : Constant  Value=false
  Equal Front Rear Bias : Selector  InputPortWidth=1  IndexOptions=Index vector (dialog)  Indices=[1 1]  OutputSizes=1
  Gain : Gain
  Hill Hold : Subsystem
  Linear Predictive Driver : vehdynlibdriver/Predictive Driver  extAccelOvr=on  extDecelOvr=on  extAccelHld=on  extDecelHld=on  extAccelZero=on  extDecelZero=on  extSteerOvr=on  extSteerHld=on  extSteerZero=on  cntrlType=Predictive  cntrlTypeLat=Predictive  shftType=Reverse, Neutral, Drive  coordMode=SAE J670 (Z-down)  refType=Reference pose  velUnits=m/s  angUnits=rad  gearOut=on  steerOut=on  Kp=3  Ki=1  Kff=1  Kg=0  VehVelVec=[0 100]  KffVec=[.1 .1]  KpVec=[10 10]  KiVec=[5 5]  KgVec=[0 0]  vnom=5  Kaw=1  tauerr=.075  tau=DriverTimeConst  L=DriverPreviewDist  Kpt=DriverTractiveForce  aR=DriverRollRes  bR=DriverDrivelineRes  cR=DriverAeroRes  g=EnvGrvty  vecPose=off  dynamMode=off  PositionGainF=2.5  PositionGainR=2.5  YawRateGain=.2  DelayGain=.2  enableDrift=off  BetaRef=10  KpBeta=1  KpDrift=1  KdDrift=1  KpPsi=1  KOmega=.1  tOmega=.1  a=MotoFrmLngth  b=MotoRearArmLngth  m=MotoFrmMass+MotoUpprFrntFrkMass+MotoLowrFrntFrkMass+MotoRearArmMass+RiderMass  Cy_f=DriverFrontCornerStiff  Cy_r=DriverRearCornerStiff  I=MotoFrmInert(3)  Ksteer=1  theta=DriverWheelRange  Idl=1  Re=PlntWhlLdRadius  lambda_mu=1  GearInit=DriverInitialGear  tShift=DriverShiftTime  pdlVec=[0.1 0.4 0.5 0.9]  upShftTbl=[-1 12.9375 26.4375 39.9375 51.18749999999999 62.4375 72.84375 83.25;-1 16.3125 29.8125 43.3125 54.5624 65.8125 76.78125 87.75;-1 19.6875 33.1875 46.68749999999999 57.9375 69.1875 80.71875 92.25;-1 33 52.5 77.25 100.5 138.75 161.875 185]  dwnShftTbl=[-1 12.9375 26.4375 39.9375 51.18749999999999 62.4375 72.84375 83.25;-1 16.3125 29.8125 43.3125 54.5624 65.8125 76.78125 87.75;-1 19.6875 33.1875 46.68749999999999 57.9375 69.1875 80.71875 92.25;-1 33 52.5 77.25 100.5 138.75 161.875 185]  tClutch=.5  tRev=.5  tPark=120  UpGearVec="[0  1  2  3  4  5  6  7]"  DownGearVec="[1  2  3  4  5  6  7  8]"  aMode=2
  Signal Specification4 : SignalSpecification  Unit=N*m
  Terminator : Terminator
  Unit Conversion : UnitConversion
  " Rider" : Outport  VectorParamsAs1DForOutWhenUnconnected=off
  wires:
  Linear Predictive Driver/3 -> Bus Creator1/2  "AccelCmd"
  Bus Selector/2 -> Linear Predictive Driver/18  "<ydot>"
  Bus Selector/1 -> Linear Predictive Driver/17  "<Y>"
  Bus Selector1/10 -> Linear Predictive Driver/10  "<AccelZero>"
  Bus Creator1/1 -> " Rider"/1
  Linear Predictive Driver/1 -> Terminator/1
  Bus Selector/3 -> Linear Predictive Driver/19  "<psi>"
  MotoFdbk/1 -> Hill Hold/7(VehFdbk), Bus Selector/1
  Bus Selector1/2 -> Linear Predictive Driver/2  "<LtrlRef>"
  Bus Selector/4 -> Linear Predictive Driver/20  "<r>"
  MotoRef/1 -> Bus Selector1/1
  Bus Selector1/1 -> Unit Conversion/1  "<LngRef>"
  Signal Specification4/1 -> Bus Creator1/1  "SteerCmd"
  Linear Predictive Driver/4 -> Equal Front Rear Bias/1  "DecelCmd"
  Linear Predictive Driver/5 -> Bus Creator1/4  "GearCmd"
  Constant/1 -> Bus Creator1/5  "IgnSwtch"
  Bus Selector1/3 -> Linear Predictive Driver/3  "<EnblSteerCmd>"
  Bus Selector1/4 -> Linear Predictive Driver/4  "<SteerOvrCmd>"
  Bus Selector1/5 -> Linear Predictive Driver/5  "<SteerHld>"
  Bus Selector1/6 -> Linear Predictive Driver/6  "<SteerZero>"
  Bus Selector1/7 -> Linear Predictive Driver/7  "<EnblAccelOvr>"
  Bus Selector1/8 -> Linear Predictive Driver/8  "<AccelOvrCmd>"
  Bus Selector1/9 -> Linear Predictive Driver/9  "<AccelHld>"
  Bus Selector1/11 -> Hill Hold/2(<EnblDecelCmd>)  "<EnblDecelCmd>"
  Bus Selector1/12 -> Hill Hold/3(<DecelOvrCmd>)  "<DecelOvrCmd>"
  Bus Selector1/13 -> Hill Hold/4(<DecelHld>)  "<DecelHld>"
  Bus Selector1/14 -> Hill Hold/5(<DecelZero>)  "<DecelZero>"
  Env/1 -> Hill Hold/6(Env)
  Hill Hold/5(Grade) -> Linear Predictive Driver/15
  Hill Hold/6(VelFdbk) -> Linear Predictive Driver/16
  Hill Hold/4(DecelZero) -> Linear Predictive Driver/14
  Hill Hold/3(DecelHld) -> Linear Predictive Driver/13
  Hill Hold/2(DecelOvrCmd) -> Linear Predictive Driver/12
  Hill Hold/1(EnblDecelOvr) -> Linear Predictive Driver/11
  Unit Conversion/1 -> Linear Predictive Driver/1, Hill Hold/1(LngRef)
  Equal Front Rear Bias/1 -> Bus Creator1/3  "DecelCmd"
  Gain/1 -> Signal Specification4/1
  Linear Predictive Driver/2 -> Gain/1  "SteerCmd"

== system VirtualMotoTemplate/Rider Commands/Rider Commands/Predictive Stanley Rider ==
  MotoRef : Inport
  MotoFdbk : Inport  Port=2
  Env : Inport  Port=3
  Bus Creator1 : BusCreator  Inputs=5
  Bus Selector : BusSelector  OutputSignals=Body.InertFrm.Cg.Disp.X,Body.InertFrm.Cg.Disp.Y,Body.InertFrm.Cg.Ang.psi
  Bus Selector1 : BusSelector  OutputSignals=LngRef,PoseRef,EnblSteerCmd,SteerOvrCmd,SteerHld,SteerZero,EnblAccelOvr,AccelOvrCmd,AccelHld,AccelZero,EnblDecelCmd,DecelOvrCmd,DecelHld,DecelZero,CurvRef
  Constant : Constant  Value=false
  Equal Front Rear Bias : Selector  InputPortWidth=1  IndexOptions=Index vector (dialog)  Indices=[1 1]  OutputSizes=1
  Gain : Gain
  Hill Hold : Subsystem
  Linear Predictive Driver : vehdynlibdriver/Predictive Driver  extAccelOvr=on  extDecelOvr=on  extAccelHld=on  extDecelHld=on  extAccelZero=on  extDecelZero=on  extSteerOvr=on  extSteerHld=on  extSteerZero=on  cntrlType=Predictive  cntrlTypeLat=Stanley  shftType=Reverse, Neutral, Drive  coordMode=SAE J670 (Z-down)  refType=Reference pose  velUnits=m/s  angUnits=rad  gearOut=on  steerOut=on  Kp=3  Ki=1  Kff=1  Kg=0  VehVelVec=[0 100]  KffVec=[.1 .1]  KpVec=[10 10]  KiVec=[5 5]  KgVec=[0 0]  vnom=5  Kaw=1  tauerr=.075  tau=DriverTimeConst  L=DriverPreviewDist  Kpt=DriverTractiveForce  aR=DriverRollRes  bR=DriverDrivelineRes  cR=DriverAeroRes  g=EnvGrvty  vecPose=on  dynamMode=off  PositionGainF=2.5  PositionGainR=2.5  YawRateGain=.2  DelayGain=.2  enableDrift=off  BetaRef=10  KpBeta=1  KpDrift=1  KdDrift=1  KpPsi=1  KOmega=.1  tOmega=.1  a=MotoFrmLngth  b=MotoRearArmLngth  m=MotoFrmMass+MotoUpprFrntFrkMass+MotoLowrFrntFrkMass+MotoRearArmMass+RiderMass  Cy_f=DriverFrontCornerStiff  Cy_r=DriverRearCornerStiff  I=MotoFrmInert(3)  Ksteer=1  theta=DriverWheelRange  Idl=1  Re=PlntWhlLdRadius  lambda_mu=1  GearInit=DriverInitialGear  tShift=DriverShiftTime  pdlVec=[0.1 0.4 0.5 0.9]  upShftTbl=[-1 12.9375 26.4375 39.9375 51.18749999999999 62.4375 72.84375 83.25;-1 16.3125 29.8125 43.3125 54.5624 65.8125 76.78125 87.75;-1 19.6875 33.1875 46.68749999999999 57.9375 69.1875 80.71875 92.25;-1 33 52.5 77.25 100.5 138.75 161.875 185]  dwnShftTbl=[-1 12.9375 26.4375 39.9375 51.18749999999999 62.4375 72.84375 83.25;-1 16.3125 29.8125 43.3125 54.5624 65.8125 76.78125 87.75;-1 19.6875 33.1875 46.68749999999999 57.9375 69.1875 80.71875 92.25;-1 33 52.5 77.25 100.5 138.75 161.875 185]  tClutch=.5  tRev=.5  tPark=120  UpGearVec="[0  1  2  3  4  5  6  7]"  DownGearVec="[1  2  3  4  5  6  7  8]"  aMode=2
  Mux : Mux  Inputs=3
  Signal Specification4 : SignalSpecification  Unit=N*m
  Terminator : Terminator
  Unit Conversion : UnitConversion
  " Rider" : Outport  VectorParamsAs1DForOutWhenUnconnected=off
  wires:
  Unit Conversion/1 -> Hill Hold/1(LngRef), Linear Predictive Driver/1
  Hill Hold/1(EnblDecelOvr) -> Linear Predictive Driver/11
  Hill Hold/2(DecelOvrCmd) -> Linear Predictive Driver/12
  Hill Hold/3(DecelHld) -> Linear Predictive Driver/13
  Hill Hold/4(DecelZero) -> Linear Predictive Driver/14
  Hill Hold/6(VelFdbk) -> Linear Predictive Driver/16
  Hill Hold/5(Grade) -> Linear Predictive Driver/15
  Env/1 -> Hill Hold/7(Env)
  Bus Selector1/14 -> Hill Hold/5(<DecelZero>)  "<DecelZero>"
  Bus Selector1/13 -> Hill Hold/4(<DecelHld>)  "<DecelHld>"
  Bus Selector1/12 -> Hill Hold/3(<DecelOvrCmd>)  "<DecelOvrCmd>"
  Bus Selector1/11 -> Hill Hold/2(<EnblDecelCmd>)  "<EnblDecelCmd>"
  Bus Selector1/9 -> Linear Predictive Driver/9  "<AccelHld>"
  Bus Selector1/8 -> Linear Predictive Driver/8  "<AccelOvrCmd>"
  Bus Selector1/7 -> Linear Predictive Driver/7  "<EnblAccelOvr>"
  Bus Selector1/6 -> Linear Predictive Driver/6  "<SteerZero>"
  Bus Selector1/5 -> Linear Predictive Driver/5  "<SteerHld>"
  Bus Selector1/4 -> Linear Predictive Driver/4  "<SteerOvrCmd>"
  Bus Selector1/3 -> Linear Predictive Driver/3  "<EnblSteerCmd>"
  Constant/1 -> Bus Creator1/5  "IgnSwtch"
  Linear Predictive Driver/5 -> Bus Creator1/4  "GearCmd"
  Linear Predictive Driver/4 -> Equal Front Rear Bias/1  "DecelCmd"
  Signal Specification4/1 -> Bus Creator1/1  "SteerCmd"
  Bus Selector1/1 -> Unit Conversion/1  "<LngRef>"
  MotoRef/1 -> Bus Selector1/1
  Bus Selector1/2 -> Linear Predictive Driver/2  "<PoseRef>"
  MotoFdbk/1 -> Hill Hold/8(VehFdbk), Bus Selector/1
  Linear Predictive Driver/1 -> Terminator/1
  Bus Creator1/1 -> " Rider"/1
  Bus Selector1/10 -> Linear Predictive Driver/10  "<AccelZero>"
  Linear Predictive Driver/3 -> Bus Creator1/2  "AccelCmd"
  Bus Selector1/15 -> Hill Hold/6(<CurvRef>)  "<CurvRef>"
  Bus Selector/3 -> Mux/3  "<psi>"
  Bus Selector/1 -> Mux/1  "<X>"
  Bus Selector/2 -> Mux/2  "<Y>"
  Mux/1 -> Linear Predictive Driver/17
  Equal Front Rear Bias/1 -> Bus Creator1/3  "DecelCmd"
  Gain/1 -> Signal Specification4/1
  Linear Predictive Driver/2 -> Gain/1  "SteerCmd"
